simulink model "QuadrotorSimulink_w_memory"  (R2020a)
settings: Solver=FixedStepAuto  StartTime=0.0  StopTime=options.T_train  FixedStep=0.001  RelTol=1e-6
undefined symbols (not defined in the file or in its folder): options, Quad
libraries: neural x134, simulink x2
(part 5 of 8)

== system QuadrotorSimulink_w_memory/NN/Layer 3/Delays 1 ==
  "p{3}" : Inport  PortDimensions=30
      mask Display: e = 0.06;c1 = [120 230 180]/255;c2 = ([120 230 180]+0)/(256+128);c3 = ([120 230 180]+128)/(256+128);patch([0 1 1 0],[0 0 1 1],c1);patch([0 1 1 1-e 1-e 0+e],[0 0 1 1-e 0+e 0+e],c2);patch([0 0 1 1-e 0+e 0+e],[0 1 1 1-e 1-e 0+e],c3);plot([0 1 1 0 0],[0 0 1 1 0]);
  mux : Mux  Inputs=1
      mask Display: e = 0.06;c1 = [120 150 230]/255;c2 = ([120 150 230]+0)/383;c3 = ([120 150 230]+128)/383;patch([0 1 1 0],[0 0 1 1],c1);patch([0 1 1 1-e 1-e 0+e],[0 0 1 1-e 0+e 0+e],c2);patch([0 0 1 1-e 0+e 0+e],[0 1 1 1-e 1-e 0+e],c3);plot([0 1 1 0 0],[0 0 1 1 0]);disp('Mux')
  "pd{3,2}" : Outport
      mask Display: e = 0.06;c1 = [120 230 180]/255;c2 = ([120 230 180]+0)/(256+128);c3 = ([120 230 180]+128)/(256+128);patch([0 1 1 0],[0 0 1 1],c1);patch([0 1 1 1-e 1-e 0+e],[0 0 1 1-e 0+e 0+e],c2);patch([0 0 1 1-e 0+e 0+e],[0 1 1 1-e 1-e 0+e],c3);plot([0 1 1 0 0],[0 0 1 1 0]);
  wires:
  "p{3}"/1 -> mux/1
  mux/1 -> "pd{3,2}"/1

== system QuadrotorSimulink_w_memory/NN/Layer 3/LW{3,2} ==
  "ad{3,2}" : Inport  PortDimensions=30
      mask Display: e = 0.06;c1 = [120 230 180]/255;c2 = ([120 230 180]+0)/(256+128);c3 = ([120 230 180]+128)/(256+128);patch([0 1 1 0],[0 0 1 1],c1);patch([0 1 1 1-e 1-e 0+e],[0 0 1 1-e 0+e 0+e],c2);patch([0 0 1 1-e 0+e 0+e],[0 1 1 1-e 1-e 0+e],c3);plot([0 1 1 0 0],[0 0 1 1 0]);
  "IW{3,2}(1,:)'" : Constant  Value=[-1.2377658212754008015821227672859095036983489990234375;1.3313379546965025124194426098256371915340423583984375;0.8352944335663992081464357397635467350482940673828125;-0.62872309768726208911715502836159430444240570068359375;-2.136244992824471555792342769564129412174224853515625;-1.18292700822326413145901824464090168476104736328125;0.672500848051803767901901665027253329753875732421875;-0.09445194123984775036451111418500659056007862091064453125;1.372070435982643221706211988930590450763702392578125;1.8837196962722397852729727674159221351146697998046875;1.2291147804582462921274554901174269616603851318359375;0.2149422544427838366321026342120603658258914947509765625;-0.70889336803441416190452173395897261798381805419921875;-0.324295066811605303680465794968768022954463958740234375;-0.970863070871580635667896785889752209186553955078125;-0.82755296216108298335001336454297415912151336669921875;0.446012588876417204186708431734587065875530242919921875;0.254403566995133834094389158053672872483730316162109375;-0.2061566986065682394180242908987565897405147552490234375;-0.34813114631558683687018174168770201504230499267578125;0.82109841308245368196594426990486681461334228515625;1.3875041596676049859837576150312088429927825927734375;1.3184932807783720232208679590257816016674041748046875;0.3741576688360364055796480897697620093822479248046875;0.67780919814352402763546479036449454724788665771484375;0.571874880076741920476024461095221340656280517578125;-0.689821511929984421129802285577170550823211669921875;-1.3997439740832515742141595183056779205799102783203125;0.194941207079834144533236894858418963849544525146484375;0.56304853353989159359116456471383571624755859375]
      mask Display: e = 0.06;c1 = [120 150 230]/255;c2 = ([120 150 230]+0)/383;c3 = ([120 150 230]+128)/383;patch([0 1 1 0],[0 0 1 1],c1);patch([0 1 1 1-e 1-e 0+e],[0 0 1 1-e 0+e 0+e],c2);patch([0 0 1 1-e 0+e 0+e],[0 1 1 1-e 1-e 0+e],c3);plot([0 1 1 0 0],[0 0 1 1 0]);disp('weights');
  "IW{3,2}(2,:)'" : Constant  Value=[0.5195890680643799885984890352119691669940948486328125;-0.6168600450060097717397411543061025440692901611328125;-0.665659817113567253699102366226725280284881591796875;-0.711577668427772369597050783340819180011749267578125;0.81463815413262263831484233378432691097259521484375;0.137373376990872875236249228692031465470790863037109375;0.81953990245624519506151273162686266005039215087890625;-0.770324358175269896520376278203912079334259033203125;-0.31343183693245679766192779425182379782199859619140625;-0.322037144731480207138218929685535840690135955810546875;0.7724765917313376473174457714776508510112762451171875;0.028200965523960459802044198340809089131653308868408203125;0.30360193552423897500602834043093025684356689453125;0.14339021560964237966828704884392209351062774658203125;-0.65463193034585620555532159414724446833133697509765625;-0.537680726635834549398396120523102581501007080078125;-0.05041648879177403064222318107567843981087207794189453125;0.355130294580800087711480728103197179734706878662109375;0.293944508490420697288669771296554245054721832275390625;0.8409620519632377000363021579687483608722686767578125;-0.379736562836066215975705517848837189376354217529296875;-0.92502371867099142388468635544995777308940887451171875;0.11414153388485810680652576820648391731083393096923828125;0.29309959291450160545622338759130798280239105224609375;-0.8121424240890668944103936155443079769611358642578125;-1.0947438828232083363189985902863554656505584716796875;0.99591487667312061926594424221548251807689666748046875;0.2163678340176413417150769191721337847411632537841796875;-0.64319933541768536944260858945199288427829742431640625;0.80413412660001981624446898422320373356342315673828125]
      mask Display: e = 0.06;c1 = [120 150 230]/255;c2 = ([120 150 230]+0)/383;c3 = ([120 150 230]+128)/383;patch([0 1 1 0],[0 0 1 1],c1);patch([0 1 1 1-e 1-e 0+e],[0 0 1 1-e 0+e 0+e],c2);patch([0 0 1 1-e 0+e 0+e],[0 1 1 1-e 1-e 0+e],c3);plot([0 1 1 0 0],[0 0 1 1 0]);disp('weights');
  Mux : Mux  Inputs=2
      mask Display: e = 0.06;c1 = [120 150 230]/255;c2 = ([120 150 230]+0)/383;c3 = ([120 150 230]+128)/383;patch([0 1 1 0],[0 0 1 1],c1);patch([0 1 1 1-e 1-e 0+e],[0 0 1 1-e 0+e 0+e],c2);patch([0 0 1 1-e 0+e 0+e],[0 1 1 1-e 1-e 0+e],c3);plot([0 1 1 0 0],[0 0 1 1 0]);disp('Mux');
  dotprod1 : neural/Weight Functions/dotprod
  dotprod2 : neural/Weight Functions/dotprod
  "lz{3,2}" : Outport
      mask Display: e = 0.06;c1 = [120 230 180]/255;c2 = ([120 230 180]+0)/(256+128);c3 = ([120 230 180]+128)/(256+128);patch([0 1 1 0],[0 0 1 1],c1);patch([0 1 1 1-e 1-e 0+e],[0 0 1 1-e 0+e 0+e],c2);patch([0 0 1 1-e 0+e 0+e],[0 1 1 1-e 1-e 0+e],c3);plot([0 1 1 0 0],[0 0 1 1 0]);
  wires:
  "IW{3,2}(1,:)'"/1 -> dotprod1/1
  "ad{3,2}"/1 -> dotprod1/2, dotprod2/2
  dotprod1/1 -> Mux/1
  "IW{3,2}(2,:)'"/1 -> dotprod2/1
  dotprod2/1 -> Mux/2
  Mux/1 -> "lz{3,2}"/1

== system QuadrotorSimulink_w_memory/NN_online/Layer 1/Delays 1 ==
  "p{1}" : Inport  PortDimensions=20
      mask Display: e = 0.06;c1 = [120 230 180]/255;c2 = ([120 230 180]+0)/(256+128);c3 = ([120 230 180]+128)/(256+128);patch([0 1 1 0],[0 0 1 1],c1);patch([0 1 1 1-e 1-e 0+e],[0 0 1 1-e 0+e 0+e],c2);patch([0 0 1 1-e 0+e 0+e],[0 1 1 1-e 1-e 0+e],c3);plot([0 1 1 0 0],[0 0 1 1 0]);
  mux : Mux  Inputs=1
      mask Display: e = 0.06;c1 = [120 150 230]/255;c2 = ([120 150 230]+0)/383;c3 = ([120 150 230]+128)/383;patch([0 1 1 0],[0 0 1 1],c1);patch([0 1 1 1-e 1-e 0+e],[0 0 1 1-e 0+e 0+e],c2);patch([0 0 1 1-e 0+e 0+e],[0 1 1 1-e 1-e 0+e],c3);plot([0 1 1 0 0],[0 0 1 1 0]);disp('Mux')
  "pd{1,1}" : Outport
      mask Display: e = 0.06;c1 = [120 230 180]/255;c2 = ([120 230 180]+0)/(256+128);c3 = ([120 230 180]+128)/(256+128);patch([0 1 1 0],[0 0 1 1],c1);patch([0 1 1 1-e 1-e 0+e],[0 0 1 1-e 0+e 0+e],c2);patch([0 0 1 1-e 0+e 0+e],[0 1 1 1-e 1-e 0+e],c3);plot([0 1 1 0 0],[0 0 1 1 0]);
  wires:
  "p{1}"/1 -> mux/1
  mux/1 -> "pd{1,1}"/1
